simulink model "Final_Q1_D_end"  (R2019a)
settings: Solver=VariableStepAuto  StartTime=0.0  StopTime=60.0  RelTol=1e-3
libraries: simulink x1
settings Model: Creator=kullanıcı  LastModifiedBy=hp

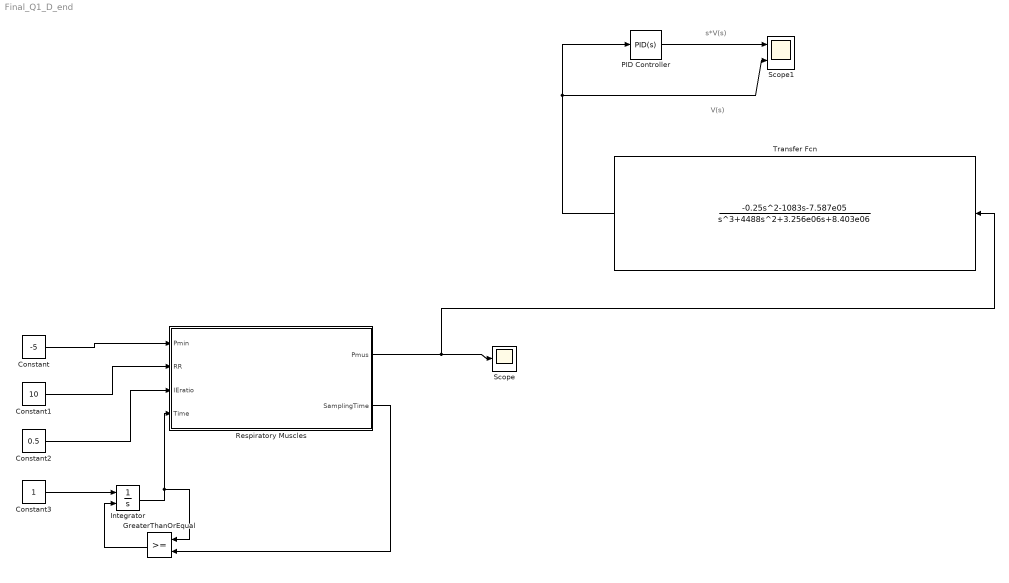
== system Final_Q1_D_end ==
  note: V(s)
  note: s*V(s)
  Constant : Constant  Value=-5
  Constant1 : Constant  Value=10
  Constant2 : Constant  Value=0.5
  Constant3 : Constant
  GreaterThanOrEqual : RelationalOperator  OutDataTypeStr=boolean  RndMeth=Simplest
  Integrator : Integrator  ExternalReset=rising
  PID Controller : simulink/Continuous/PID Controller  Controller=PID  Form=Parallel  TimeDomain=Continuous-time  SampleTime=-1  IntegratorMethod=Forward Euler  FilterMethod=Forward Euler  ControllerParametersSource=internal  P=0  I=0  D=1  UseFilter=on  N=100  TunerSelectOption=Transfer Function Based (PID Tuner App)  InitialConditionSource=internal  InitialConditionForIntegrator=0  InitialConditionForFilter=0  DifferentiatorICPrevScaledInput=0  ExternalReset=none  TrackingMode=off  Kt=1  LimitOutput=off  UpperSaturationLimit=inf  LowerSaturationLimit=-inf  LinearizeAsGain=on  AntiWindupMode=none  Kb=1  POutMin=[]  POutMax=[]  IOutMin=[]  IOutMax=[]  DOutMin=[]  DOutMax=[]  NOutMin=[]  NOutMax=[]  SumOutMin=[]  SumOutMax=[]  SaturationOutMin=[]  SaturationOutMax=[]  PParamMin=[]  PParamMax=[]  IParamMin=[]  IParamMax=[]  DParamMin=[]  DParamMax=[]  NParamMin=[]  NParamMax=[]  KbParamMin=[]  KbParamMax=[]  KtParamMin=[]  KtParamMax=[]  KbOutMin=[]  KbOutMax=[]  KtOutMin=[]  KtOutMax=[]  IntegratorOutMin=[]  IntegratorOutMax=[]  FilterOutMin=[]  FilterOutMax=[]  SumI1OutMin=[]  SumI1OutMax=[]  SumI2OutMin=[]  SumI2OutMax=[]  SumI3OutMin=[]  SumI3OutMax=[]  SumI4OutMin=[]  SumI4OutMax=[]  SumDOutMin=[]  SumDOutMax=[]  DifferentiatorOutMin=[]  DifferentiatorOutMax=[]  FilterDiffOutCoefMin=[]  FilterDiffOutCoefMax=[]  ReciprocalOutMin=[]  ReciprocalOutMax=[]  SumDenOutMin=[]  SumDenOutMax=[]  SumNumOutMin=[]  SumNumOutMax=[]  DivideOutMin=[]  DivideOutMax=[]  IntegratorContinuousStateAttributes=''  IntegratorStateMustResolveToSignalObject=off  IntegratorRTWStateStorageClass=Auto  FilterContinuousStateAttributes=''  FilterStateMustResolveToSignalObject=off  FilterRTWStateStorageClass=Auto  ParallelPVariant=InternalParameters  IdealPVariant=Disabled  IVariant=InternalParameters  DVariant=InternalParameters  IntegratorVariant=Continuous  SatVariant=Disabled  AWVariant=Passthrough  PCopyVariant=Disabled  TRVariant=Disabled  FdbkBlocksVariant=Forward  IdealPFdbkVariant=Disabled  SatFdbkVariant=Disabled  DerivativeFilterVariant=ContFilter  NVariant=InternalParameters  NCopyVariant=Disabled  FilterICVariant=InternalICsFilter  IntegratorICVariant=InternalICs  ExternalResetVariant=Disabled  TRSumVariant=Passthrough  SumFdbkVariant=Disabled  SumVariant=Sum_PID
  Respiratory Muscles : MATLAB Function  TreatAsAtomicUnit=on
  Scope : Scope
  Scope1 : Scope  NumInputPorts=2
  Transfer Fcn : TransferFcn  Numerator=[-0.25 -1083 -7.587e05]  Denominator=[1 4488 3.256e06 8.403e06]
  wires:
  GreaterThanOrEqual/1 -> Integrator/2
  Constant1/1 -> Respiratory Muscles/2(RR)
  PID Controller/1 -> Scope1/1
  Constant2/1 -> Respiratory Muscles/3(IEratio)
  Respiratory Muscles/2(SamplingTime) -> GreaterThanOrEqual/2
  Respiratory Muscles/1(Pmus) -> Transfer Fcn/1, Scope/1
  Transfer Fcn/1 -> PID Controller/1, Scope1/2
  Integrator/1 -> Respiratory Muscles/4(Time), GreaterThanOrEqual/1
  Constant3/1 -> Integrator/1
  Constant/1 -> Respiratory Muscles/1(Pmin)

== matlab function Final_Q1_D_end/Respiratory Muscles ==
  data: Pmin input; Pmus output; RR input; IEratio input; Time input; SamplingTime output
function [Pmus,SamplingTime] = fcn(Pmin,RR ,IEratio, Time)
T = 60/RR;
SamplingTime = T; 
TE = T/(1 + IEratio);
TI = T - TE;
Tau = TE / 10;

if (Time <= TI)

    Pmus = Pmin*(1/(TI*TE))*(T*Time -Time^2)
    

else 
    
    Pmus = (Pmin/(1 - exp((-TE/Tau))))*(exp(((Time - TI)/(-Tau)))-exp(((-TE)/(Tau))))
end


end
